simulink model "hoverSim_pid_RL"  (R2025b)
settings: Solver=ode45  StartTime=0.0  StopTime=30  RelTol=1e-3  AbsTol=1e-3  EnableMultiTasking=on
values from neighbouring files (symbols this model uses):
  A = [0 0 0 1 0 0 ... (first row only)    [setupHover.m]
  B = [0     0     0     0 ... (first row only)    [setupHover.m]
  C = [1 0 0 0 0 0 ... (first row only)    [setupHover.m]
  CMD_RATE_LIMIT = 60 * pi/180    (= 1.0471975512)    [setupHover.m]
  D = zeros(3,4)    [setupHover.m]
  K = [ 1  1  0 ... (first row only)    [setupHover.m]
  V_bias = 2.0    (= 2)    [setupHover.m]
  VMAX_AMP = 24    [setupHover.m]
  wcf = 2 * pi * 20    (= 125.663706144)    [setupHover.m]
  zetaf = 0.6    [setupHover.m]
undefined symbols (not defined in the file or in its folder): X, Y, Z
libraries: sm_lib x30, rllib x18, simulink_extras x17, slpidlib x6, nesl_utility x4, simulink x2
(part 3 of 3)

== matlab function hoverSim_pid_RL/Rate_PID/yaw_rate_pid/MATLAB Function3 ==
  data: t input; isDone output; yaw_rate_err input
function isDone = isDoneYaw(t, yaw_rate_err)
max_rate_error = 5;  % var 10, strammes inn
T_max          = 30;
isDone = 0;
if abs(yaw_rate_err) > max_rate_error
    isDone = 1;
    return;
end
if t >= T_max
    isDone = 1;
end
end

== matlab function hoverSim_pid_RL/Rate_PID/roll_rate_pid/MATLAB Function3 ==
  data: t input; isDone output; roll_rate_err input
function isDone = doneRollOffline(t, roll_rate_err)

MAX_RATE_ERROR = 5;
T_MAX          = 30;

isDone = 0;
if abs(roll_rate_err) > MAX_RATE_ERROR
    isDone = 1;
    return;
end
if t >= T_MAX
    isDone = 1;
end
end

== matlab function hoverSim_pid_RL/Rate_PID/roll_rate_pid/MATLAB Function1 ==
  data: Ki_action input; Ki output
% RL_roll_rate_i
function Ki = mapKi(Ki_action)
Ki = (Ki_action + 1)/2 * 25;
end

== matlab function hoverSim_pid_RL/Rate_PID/yaw_rate_pid/MATLAB Function1 ==
  data: Kp_action input; Kp output
function Kp = mapKp(Kp_action)
% Kp_action ∈ [-1, 1] → Kp ∈ [25, 35]
Kp = 25 + (Kp_action + 1)/2 * 10;
end

== matlab function hoverSim_pid_RL/Rate_PID/yaw_rate_pid/MATLAB Function2 ==
  data: Ki_action input; Ki output
function Ki = mapKi_yaw(Ki_action)
Ki = (Ki_action + 1)/2 * 25;
end

== matlab function hoverSim_pid_RL/Rate_PID/yaw_rate_pid/MATLAB Function4 ==
  data: Kd_action input; Kd output
% RL_yaw_rate_d
function Kd = mapKd(Kd_action)
Kd = (Kd_action + 1)/2 * 25;
end

== matlab function hoverSim_pid_RL/Rate_PID/pitch_rate_pid/MATLAB Function1 ==
  data: Kp_action input; Kp output
function Kp = mapKp_pitch(Kp_action)
% Kp_action ∈ [-1, 1] → Kp ∈ [5, 25]
Kp = 5 + (Kp_action + 1)/2 * 20;
end
